simulink model "rlsuspension"  (R2023a)
settings: Solver=VariableStepAuto  StartTime=0.0  StopTime=10  RelTol=1e-3
values from neighbouring files (symbols this model uses):
  bs = 20000    [TRAIN_DDPG.m]
  bus = 40000    [TRAIN_DDPG.m]
  ks = 430000    [TRAIN_DDPG.m]
  kus = 2440000    [TRAIN_DDPG.m]
  ms = 5333    [TRAIN_DDPG.m]
  mus = 906.5    [TRAIN_DDPG.m]
libraries: simulink x2, rllib x1
settings Model: Creator=Abdulrahman Hamdy  LastModifiedBy=Abdulrahman Hamdy

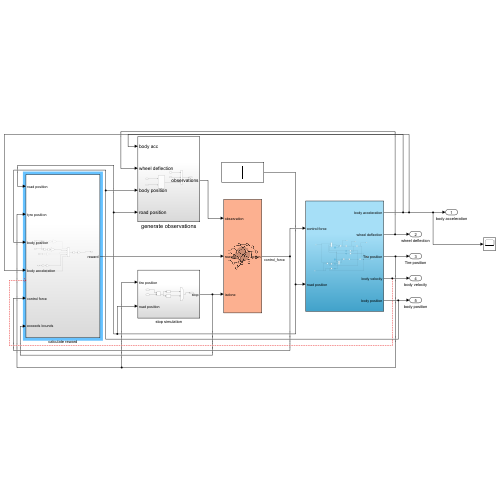
[thumbnail: Simulink's stored preview of the top-level diagram]
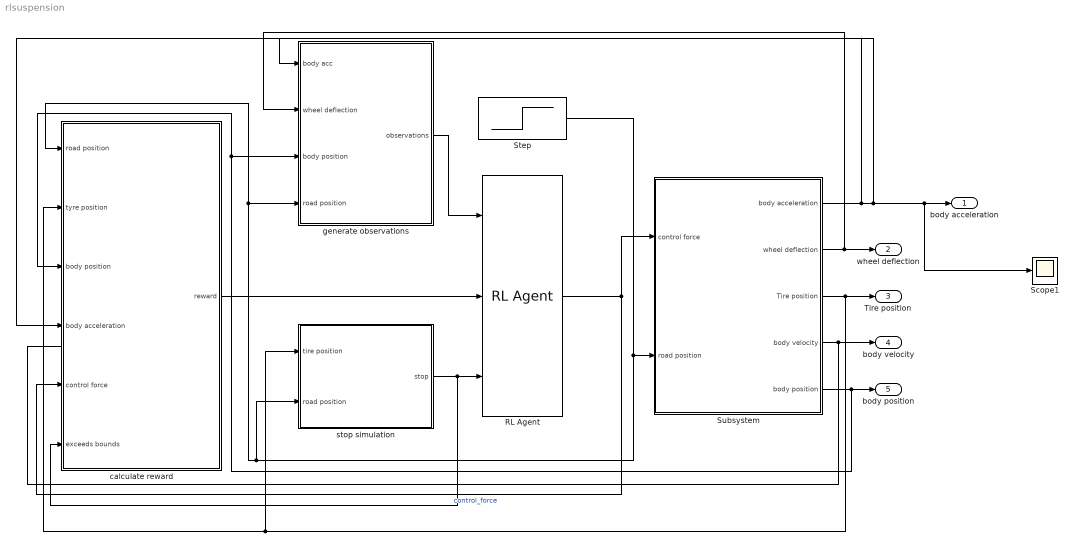
== system rlsuspension ==
  RL Agent : rllib/RL Agent  Agent=agent  ExternalActionAsInput=off  ProvideLastAction=off  ProvideCumRwd=off  TreatAsDirectFeedthrough=on  UseStrictObservationDataTypes=off
  Scope1 : Scope
  Step : Step  Time=0  SampleTime=0
  Subsystem : Subsystem
  calculate reward : Subsystem
  generate observations : Subsystem
  stop simulation : Subsystem
  body acceleration : Outport
  wheel deflection : Outport  Port=2
  Tire position : Outport  Port=3
  body velocity : Outport  Port=4
  body position : Outport  Port=5
  wires:
  stop simulation/1(stop) -> calculate reward/6(exceeds bounds), RL Agent/3
  generate observations/1(observations) -> RL Agent/1
  RL Agent/1 -> calculate reward/5(control force), Subsystem/1(control force)  "control_force"
  Subsystem/1(body acceleration) -> calculate reward/4(body acceleration), generate observations/1(body acc), Scope1/1, body acceleration/1
  Subsystem/2(wheel deflection) -> generate observations/2(wheel deflection), wheel deflection/1
  Subsystem/3(Tire position) -> stop simulation/1(tire position), calculate reward/2(tyre position), Tire position/1
  Subsystem/4(body velocity) -> body velocity/1
  Subsystem/5(body position) -> calculate reward/3(body position), generate observations/3(body position), body position/1
  Step/1 -> stop simulation/2(road position), calculate reward/1(road position), generate observations/4(road position), Subsystem/2(road position)
  calculate reward/1(reward) -> RL Agent/2

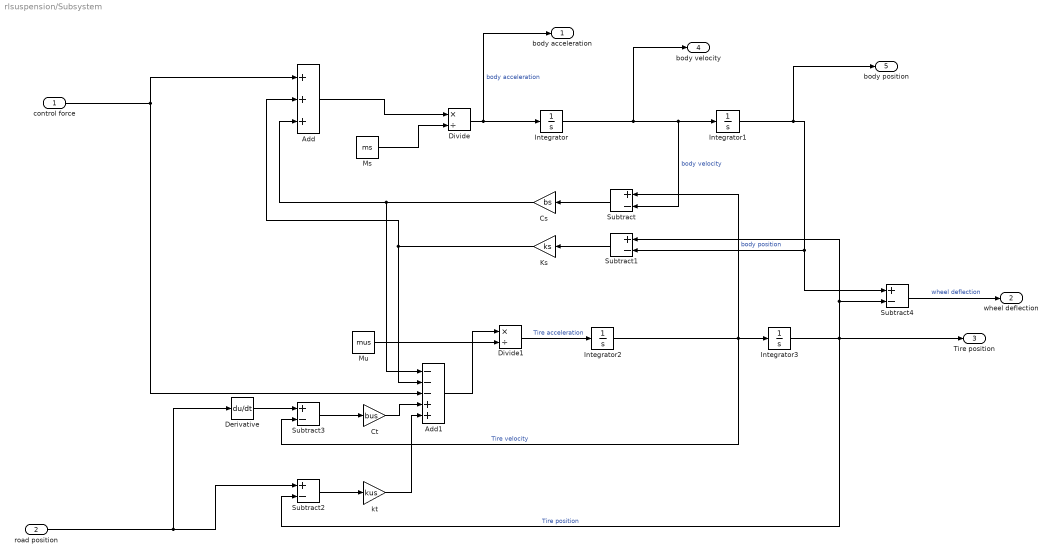
== system rlsuspension/Subsystem ==
  control force : Inport
  road position : Inport  Port=2
  Add : Sum  Inputs=+++
  Add1 : Sum  Inputs=---++
  Cs : Gain  Gain=bs
  Ct : Gain  Gain=bus
  Derivative : Derivative
  Divide : Product  Inputs=*/
  Divide1 : Product  Inputs=*/
  Integrator{,1..3} (4 alike) : Integrator
  Ks : Gain  Gain=ks
  Ms : Constant  Value=ms
  Mu : Constant  Value=mus
  Subtract{,1..4} (5 alike) : Sum  Inputs=+-
  kt : Gain  Gain=kus
  body acceleration : Outport
  wheel deflection : Outport  Port=2
  Tire position : Outport  Port=3
  body velocity : Outport  Port=4
  body position : Outport  Port=5
  wires:
  Ms/1 -> Divide/2
  Integrator1/1 -> body position/1, Subtract1/2, Subtract4/1  "body position"
  Integrator2/1 -> Subtract/1, Subtract3/2, Integrator3/1  "Tire velocity"
  Integrator3/1 -> Tire position/1, Subtract4/2, Subtract1/1, Subtract2/2  "Tire position"
  Ks/1 -> Add1/2, Add/2
  Ct/1 -> Add1/4
  Integrator/1 -> body velocity/1, Subtract/2, Integrator1/1  "body velocity"
  road position/1 -> Derivative/1, Subtract2/1
  Subtract3/1 -> Ct/1
  control force/1 -> Add1/3, Add/1
  Divide/1 -> body acceleration/1, Integrator/1  "body acceleration"
  Cs/1 -> Add1/1, Add/3
  Add1/1 -> Divide1/1
  Add/1 -> Divide/1
  kt/1 -> Add1/5
  Mu/1 -> Divide1/2
  Divide1/1 -> Integrator2/1  "Tire acceleration"
  Derivative/1 -> Subtract3/1
  Subtract1/1 -> Ks/1
  Subtract/1 -> Cs/1
  Subtract2/1 -> kt/1
  Subtract4/1 -> wheel deflection/1  "wheel deflection"

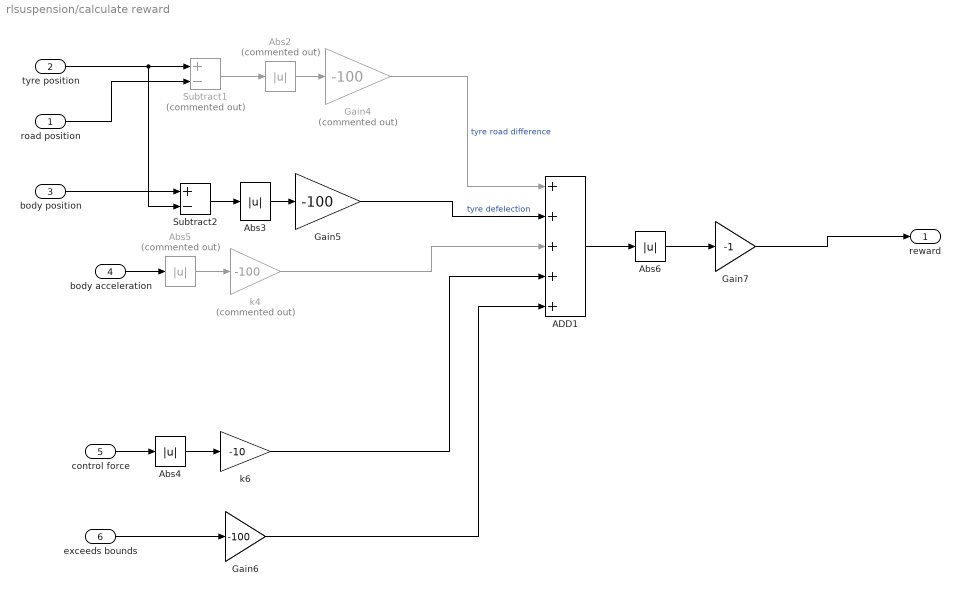
== system rlsuspension/calculate reward ==
  road position : Inport
  tyre position : Inport  Port=2
  body position : Inport  Port=3
  body acceleration : Inport  Port=4
  control force : Inport  Port=5
  exceeds bounds : Inport  Port=6
  ADD1 : Sum  Inputs=+++++
  Abs2 : Abs  Commented=on  SaturateOnIntegerOverflow=off
  Abs3 : Abs  SaturateOnIntegerOverflow=off
  Abs4 : Abs  SaturateOnIntegerOverflow=off
  Abs5 : Abs  Commented=on  SaturateOnIntegerOverflow=off
  Abs6 : Abs  SaturateOnIntegerOverflow=off
  Gain4 : Gain  Commented=on  Gain=-100
  Gain5 : Gain  Gain=-100
  Gain6 : Gain  Gain=-100
  Gain7 : Gain  Gain=-1
  Subtract1 : Sum  Commented=on  Inputs=+-
  Subtract2 : Sum  Inputs=+-
  k4 : Gain  Commented=on  Gain=-100
  k6 : Gain  Gain=-10
  reward : Outport  VectorParamsAs1DForOutWhenUnconnected=off
  wires:
  road position/1 -> Subtract1/2
  tyre position/1 -> Subtract2/2, Subtract1/1
  Subtract1/1 -> Abs2/1
  Abs2/1 -> Gain4/1
  body position/1 -> Subtract2/1
  Subtract2/1 -> Abs3/1
  Abs3/1 -> Gain5/1
  body acceleration/1 -> Abs5/1
  Abs5/1 -> k4/1
  Abs4/1 -> k6/1
  control force/1 -> Abs4/1
  Gain4/1 -> ADD1/1  "tyre road difference"
  Gain5/1 -> ADD1/2  "tyre defelection"
  k4/1 -> ADD1/3
  k6/1 -> ADD1/4
  exceeds bounds/1 -> Gain6/1
  Gain6/1 -> ADD1/5
  ADD1/1 -> Abs6/1
  Abs6/1 -> Gain7/1
  Gain7/1 -> reward/1

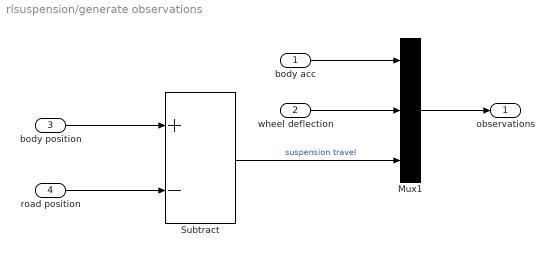
== system rlsuspension/generate observations ==
  body acc : Inport
  wheel deflection : Inport  Port=2
  body position : Inport  Port=3
  road position : Inport  Port=4
  Mux1 : Mux  Inputs=3
  Subtract : Sum  Inputs=+-
  observations : Outport  VectorParamsAs1DForOutWhenUnconnected=off
  wires:
  body acc/1 -> Mux1/1
  wheel deflection/1 -> Mux1/2
  body position/1 -> Subtract/1
  road position/1 -> Subtract/2
  Mux1/1 -> observations/1
  Subtract/1 -> Mux1/3  "suspension travel"

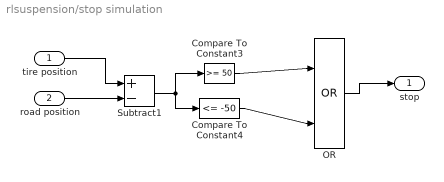
== system rlsuspension/stop simulation ==
  tire position : Inport
  road position : Inport  Port=2
  Compare To Constant3 : simulink/Logic and Bit Operations/Compare To Constant  relop=>=  const=50  OutDataTypeStr=boolean
  Compare To Constant4 : simulink/Logic and Bit Operations/Compare To Constant  relop=<=  const=-50  OutDataTypeStr=boolean
  OR : Logic  Operator=OR  IconShape=distinctive  AllPortsSameDT=off  OutDataTypeStr=boolean
  Subtract1 : Sum  Inputs=+-
  stop : Outport  VectorParamsAs1DForOutWhenUnconnected=off
  wires:
  OR/1 -> stop/1
  tire position/1 -> Subtract1/1
  Subtract1/1 -> Compare To Constant3/1, Compare To Constant4/1
  Compare To Constant3/1 -> OR/1
  road position/1 -> Subtract1/2
  Compare To Constant4/1 -> OR/2
